simulink model "slexEntityTransportDelay"  (R2024a)
settings: Solver=VariableStepAuto  StartTime=0.0  StopTime=900  RelTol=1e-3
PostLoadFcn:
  | Simulink.defineIntEnumType('OperationMode', {'Idle', 'OnDemand', 'Max'}, [0; 1; 2]);
undefined symbols (not defined in the file): m, n
Description:
  | <include>VariableSpeedConveyorBeltExample.m</include>
settings Model: PacingRate=1000  Creator=The MathWorks, Inc.  LastModifiedBy=uditpant
settings SolverCC: AlgebraicLoopSolver=TrustRegion
settings DebuggingCC: UnconnectedInputMsg=warning  UnconnectedOutputMsg=warning  UnconnectedLineMsg=warning  StrictBusMsg=ErrorOnBusTreatedAsVector  SymbolicDimsDataTypeCodeGenerationDiagnostic=none
settings ModelReferenceCC: EnableRefExpFcnMdlSchedulingChecks=on
settings RTWCC: GPUComputeCapability=3.5

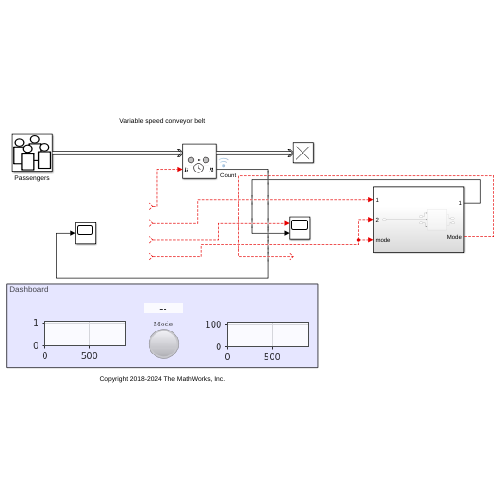
[thumbnail: Simulink's stored preview of the top-level diagram]
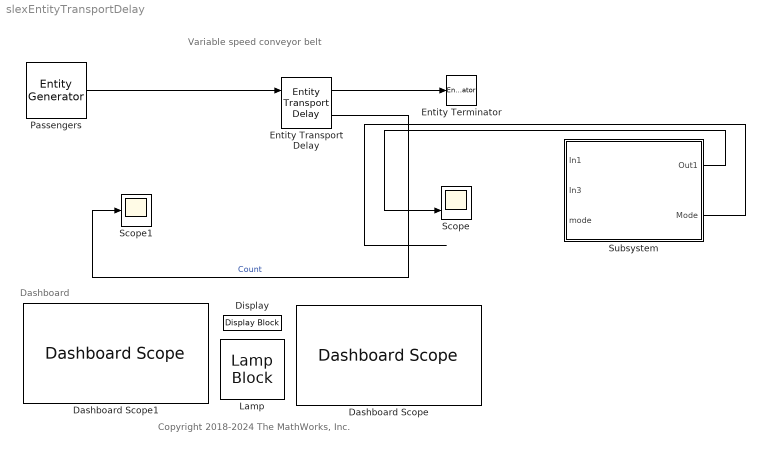
== system slexEntityTransportDelay ==
  note: Dashboard
  note: Copyright 2018-2024 The MathWorks, Inc.
  note: Variable speed conveyor belt
  Dashboard Scope : DashboardScope  Ymin=0  Ymax=110
  Dashboard Scope1 : DashboardScope  Ymin=0  Ymax=1.1000000000000001
  Display : DisplayBlock  LabelPosition=Hide  Transparency=1
  Entity Transport Delay : EntityTransportDelay  InputPortMessageModes=m,n  OutputPortMessageModes=m,n  ShowNumberEntitiesInBlock=on
  Entity Terminator : EntityTerminator  InputPortMessageModes=m
  Lamp : LampBlock
  Passengers : EntityGenerator  OutputPortMessageModes=m  TimeSource=MATLAB action  Period=0.1  IntergenerationTimeAction=|  GenerateEntityAtSimulationStart=off  EntityType=Structured  EntityTypeName=Entity
      | persistent rngInit;
      | if isempty(rngInit)
      |     seed = 12345;
      |     rng(seed);
      |     rngInit = true;
      | end
      | 
      | % Pattern: Exponential distribution
      | persistent time;
      | if isempty(time)
      |     time = 0;
      | end
      | if time < 180
      |     lambda = 2;
      | elseif time < 240
      |     lambda = .5;
      | elseif time < 300
      |     lambda = .1;
      | else
      |     time = 0;
      |     lambda = 2;
      | end
      | % Use inverse transform sampling to
      | % generate dt according to the exponential
      | % distribution
      | dt = -1/lambda * log(1 - rand());
      | time = time + dt;
      mask Display: image('$imagefile'); % Use "Edit Image" on toolstrip to change.
  Scope : Scope  NumInputPorts=2
  Scope1 : Scope
  Subsystem : Subsystem
  wires:
  Entity Transport Delay/1 -> Entity Terminator/1
  ? -> Entity Transport Delay/2
  Entity Transport Delay/2 -> Scope1/1  "Count"
  Passengers/1 -> Entity Transport Delay/1
  ? -> Subsystem/1(In1)
  ? -> Subsystem/3(mode), Subsystem/2(In3)
  Subsystem/1(Out1) -> Scope/2
  Subsystem/2(Mode) -> ?
  ? -> Scope/1

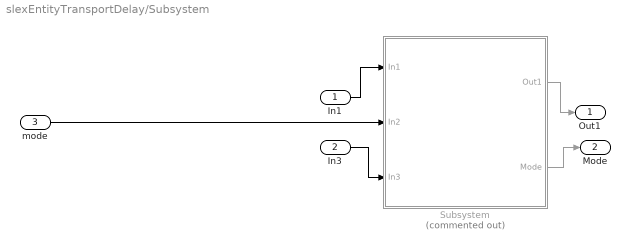
== system slexEntityTransportDelay/Subsystem ==
  In1 : Inport
  In3 : Inport  Port=2
  mode : Inport  Port=3
  Subsystem : Subsystem  Commented=on
  Out1 : Outport
  Mode : Outport  Port=2
  wires:
  In1/1 -> Subsystem/1(In1)
  mode/1 -> Subsystem/2(In2)
  In3/1 -> Subsystem/3(In3)
  Subsystem/1(Out1) -> Out1/1
  Subsystem/2(Mode) -> Mode/1

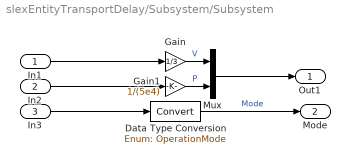
== system slexEntityTransportDelay/Subsystem/Subsystem ==
  In1 : Inport
  In2 : Inport  Port=2
  In3 : Inport  Port=3
  Data Type Conversion : DataTypeConversion  OutDataTypeStr=Enum: OperationMode  SaturateOnIntegerOverflow=off  RndMeth=Floor
  Gain : Gain  Gain=1/3
  Gain1 : Gain  Gain=1/(5e4)
  Mux : Mux  Inputs=2
  Out1 : Outport
  Mode : Outport  Port=2
  wires:
  Gain1/1 -> Mux/2  "P"
  In3/1 -> Data Type Conversion/1
  Mux/1 -> Out1/1
  Gain/1 -> Mux/1  "V"
  In1/1 -> Gain/1
  In2/1 -> Gain1/1
  Data Type Conversion/1 -> Mode/1  "Mode"
